simulink model "CanBusRagnar2020b"  (R2020b)
settings: Solver=VariableStepAuto  StartTime=0.0  StopTime=10.0  RelTol=1e-3
values from neighbouring files (symbols this model uses):
  sys_mimo = ss(A,B,C,0)    [SS_MIMO.m]
libraries: truetime x6
settings Model: Creator=mozzr  LastModifiedBy=mozzr
settings DebuggingCC: SFMachineParentedDataDiag=error

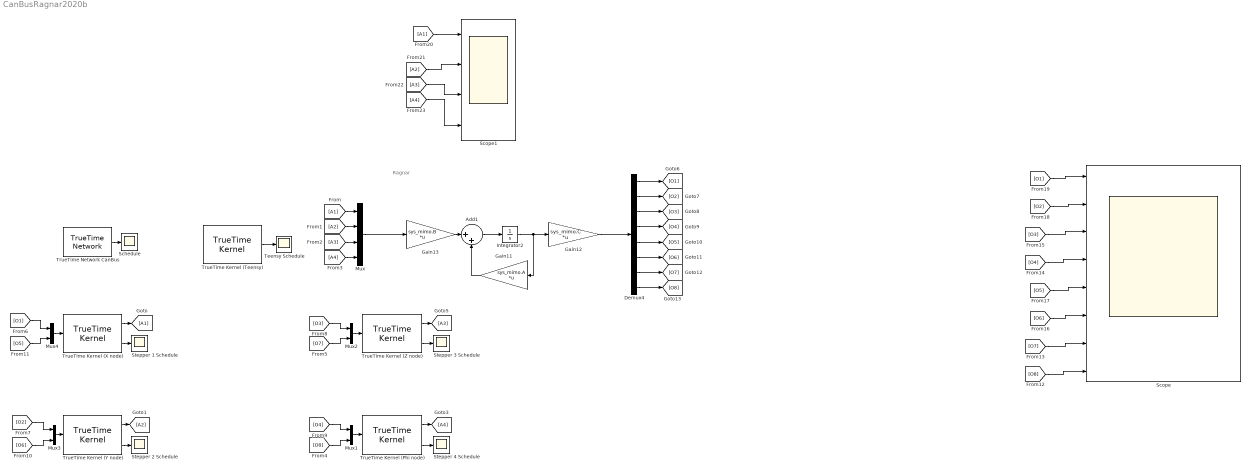
== system CanBusRagnar2020b ==
  note: Ragnar
  Add1 : Sum  Inputs=|++
  Demux4 : Demux  Outputs=8
  Gain11 : Gain  Gain=sys_mimo.A  Multiplication=Matrix(K*u)
  Gain12 : Gain  Gain=sys_mimo.C  Multiplication=Matrix(K*u)
  Gain13 : Gain  Gain=sys_mimo.B  Multiplication=Matrix(K*u)
  Integrator2 : Integrator  InitialCondition=[0 0.5 -0.4 deg2rad(90) 0 0 0 0]
  Mux : Mux
  Mux{1..4} (4 alike) : Mux  Inputs=2
  Schedule : Scope
  Scope : Scope  NumInputPorts=8
  Scope1 : Scope  NumInputPorts=4
  Stepper 1 Schedule : Scope
  Stepper 2 Schedule : Scope
  Stepper 3 Schedule : Scope
  Stepper 4 Schedule : Scope
  Teensy Schedule : Scope
  TrueTime Kernel (Phi node) : truetime/TrueTime Kernel  sfun=nodePhi_init  args=[]  ninputsoutputs=[2 1]  ntriggers=0  trigtype=falling  nwnodenbr=[1 5]  clockoffsetdrift=[0 0]  schedoutput=on  battery=off  poweroutput=off  label=1: 5
  TrueTime Kernel (Teensy) : truetime/TrueTime Kernel  sfun=Teensy_init  args=[]  ninputsoutputs=[0 0]  ntriggers=0  trigtype=falling  nwnodenbr=[1 1]  clockoffsetdrift=[0 0]  schedoutput=on  battery=off  poweroutput=off  label=1: 1
  TrueTime Kernel (X node) : truetime/TrueTime Kernel  sfun=nodeX_init  args=[]  ninputsoutputs=[2 1]  ntriggers=0  trigtype=falling  nwnodenbr=[1 2]  clockoffsetdrift=[0 0]  schedoutput=on  battery=off  poweroutput=off  label=1: 2
  TrueTime Kernel (Y node) : truetime/TrueTime Kernel  sfun=nodeY_init  args=[]  ninputsoutputs=[2 1]  ntriggers=0  trigtype=falling  nwnodenbr=[1 3]  clockoffsetdrift=[0 0]  schedoutput=on  battery=off  poweroutput=off  label=1: 3
  TrueTime Kernel (Z node) : truetime/TrueTime Kernel  sfun=nodeZ_init  args=[]  ninputsoutputs=[2 1]  ntriggers=0  trigtype=falling  nwnodenbr=[1 4]  clockoffsetdrift=[0 0]  schedoutput=on  battery=off  poweroutput=off  label=1: 4
  TrueTime Network CanBus : truetime/TrueTime Network  nwtype=CSMA/AMP (CAN)  nwnbr=1  nnodes=5  rate=10000000  minsize=512  lossprob=0  seed=0  bandwidths=[0.5 0.5]  slotsize=512  schedule=[1 1 2]  memsize=80000  buftype=Common buffer  overflow=Retransmit  dynSchedule=0  miniSlotSize=0  NIT=0  QSortMode=FIFO  sync=0  irtSchedule=0  nrtLength=0  nodeGraph=0  scheduleoutput=on
  wires:
  TrueTime Kernel (Y node)/2 -> Stepper 2 Schedule/1
  TrueTime Kernel (X node)/2 -> Stepper 1 Schedule/1
  TrueTime Kernel (Phi node)/2 -> Stepper 4 Schedule/1
  TrueTime Kernel (Z node)/2 -> Stepper 3 Schedule/1
  TrueTime Kernel (Teensy)/1 -> Teensy Schedule/1
  TrueTime Network CanBus/1 -> Schedule/1
  TrueTime Kernel (X node)/1 -> [A1]
  [A1] -> Mux/1
  TrueTime Kernel (Y node)/1 -> [A2]
  TrueTime Kernel (Phi node)/1 -> [A4]
  TrueTime Kernel (Z node)/1 -> [A3]
  [A2] -> Mux/2
  [A3] -> Mux/3
  [A4] -> Mux/4
  Demux4/1 -> [O1]
  Demux4/2 -> [O2]
  Demux4/3 -> [O3]
  Demux4/4 -> [O4]
  Demux4/5 -> [O5]
  Demux4/6 -> [O6]
  Demux4/7 -> [O7]
  Demux4/8 -> [O8]
  Mux1/1 -> TrueTime Kernel (Phi node)/1
  [O4] -> Mux1/1
  [O8] -> Mux1/2
  [O3] -> Mux2/1
  [O7] -> Mux2/2
  Mux2/1 -> TrueTime Kernel (Z node)/1
  [O2] -> Mux3/1
  [O6] -> Mux3/2
  Mux3/1 -> TrueTime Kernel (Y node)/1
  [O1] -> Mux4/1
  [O5] -> Mux4/2
  Mux4/1 -> TrueTime Kernel (X node)/1
  Gain11/1 -> Add1/2
  Gain13/1 -> Add1/1
  Add1/1 -> Integrator2/1
  Mux/1 -> Gain13/1
  Integrator2/1 -> Gain11/1, Gain12/1
  Gain12/1 -> Demux4/1
  [O8] -> Scope/8
  [O7] -> Scope/7
  [O4] -> Scope/4
  [O3] -> Scope/3
  [O5] -> Scope/5
  [O6] -> Scope/6
  [O2] -> Scope/2
  [O1] -> Scope/1
  [A1] -> Scope1/1
  [A2] -> Scope1/2
  [A3] -> Scope1/3
  [A4] -> Scope1/4
